simulink model "Quadrotor"  (R2014a)
settings: Solver=ode45  StartTime=0.0  StopTime=10.0  MaxStep=0.1  RelTol=1e-3
InitFcn:
  | parameters;
  | [b, d] = Bemt();
values from neighbouring files (symbols this model uses):
  g = 9.81    [Bemt.m]
  I = diag([0.0086,0.0086,0.0172])    [Bemt.m]
  Iprop = 12*10^-6    (= 1.2e-05)    [Bemt.m]
  Kmot = 1/(1900/60*2*pi)    (= 0.00502594557132)    [Bemt.m]
  L = 0.225    [Bemt.m]
  m = 0.58    [Bemt.m]
  Rmot = 0.128    [Bemt.m]
undefined symbols (not defined in the file or in its folder): attitudeInit, b, d, MotorSpeedInit, omegaInit, posInit, velInit
settings Model: Creator=rudink  LastModifiedBy=daniel
settings DebuggingCC: UnderspecifiedInitializationDetection=Classic  StateNameClashWarn=warning

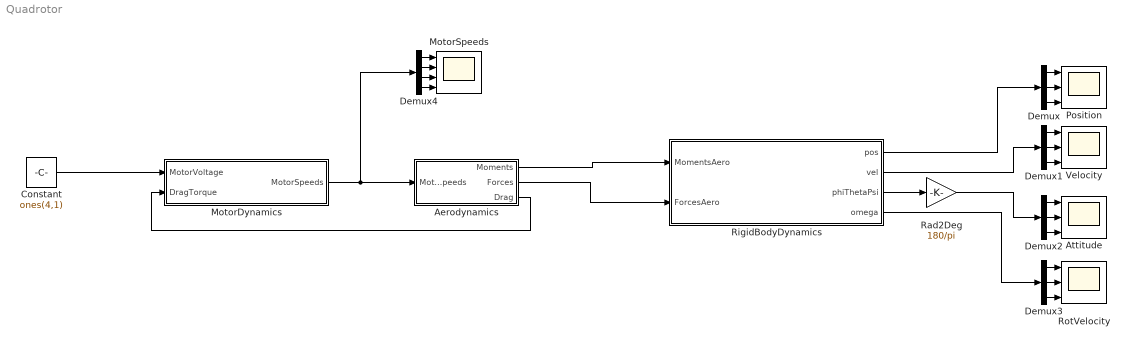
== system Quadrotor ==
  Aerodynamics : Subsystem
  Attitude : Scope  NumInputPorts=3
      settings: YMin=-5~-5~-5  YMax=5~5~5  SaveName=ScopeData2  MaxDataPoints=10000
  Constant : Constant  Value=ones(4,1)
  Demux{,1..3} (4 alike) : Demux  Outputs=3
  Demux4 : Demux
  MotorDynamics : Subsystem
  MotorSpeeds : Scope  NumInputPorts=4
      settings: YMin=-5~-5~-5~-5  YMax=5~5~5~5  SaveName=ScopeData4  MaxDataPoints=10000
  Position : Scope  NumInputPorts=3
      settings: YMin=-5~-5~-5  YMax=5~5~5  MaxDataPoints=10000
  Rad2Deg : Gain  Gain=180/pi
  RigidBodyDynamics : Subsystem
  RotVelocity : Scope  NumInputPorts=3
      settings: YMin=-5~-5~-5  YMax=5~5~5  SaveName=ScopeData3  MaxDataPoints=10000
  Velocity : Scope  NumInputPorts=3
      settings: YMin=-5~-5~-5  YMax=5~5~5  MaxDataPoints=10000
  wires:
  Demux/2 -> Position/2
  Demux/3 -> Position/3
  Demux/1 -> Position/1
  RigidBodyDynamics/1(pos) -> Demux/1
  Demux1/2 -> Velocity/2
  Demux1/3 -> Velocity/3
  Demux1/1 -> Velocity/1
  Demux2/2 -> Attitude/2
  Demux2/3 -> Attitude/3
  Demux2/1 -> Attitude/1
  Demux3/2 -> RotVelocity/2
  Demux3/3 -> RotVelocity/3
  Demux3/1 -> RotVelocity/1
  RigidBodyDynamics/2(vel) -> Demux1/1
  RigidBodyDynamics/3(phiThetaPsi) -> Rad2Deg/1
  RigidBodyDynamics/4(omega) -> Demux3/1
  Aerodynamics/2(Forces) -> RigidBodyDynamics/2(ForcesAero)
  Aerodynamics/1(Moments) -> RigidBodyDynamics/1(MomentsAero)
  Rad2Deg/1 -> Demux2/1
  MotorDynamics/1(MotorSpeeds) -> Demux4/1, Aerodynamics/1(MotorSpeeds)
  Aerodynamics/3(Drag) -> MotorDynamics/2(DragTorque)
  Constant/1 -> MotorDynamics/1(MotorVoltage)
  Demux4/2 -> MotorSpeeds/2
  Demux4/1 -> MotorSpeeds/1
  Demux4/3 -> MotorSpeeds/3
  Demux4/4 -> MotorSpeeds/4

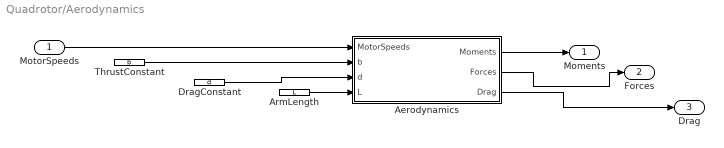
== system Quadrotor/Aerodynamics ==
  MotorSpeeds : Inport
  Aerodynamics : MATLAB Function  TreatAsAtomicUnit=on
  ArmLength : Constant  Value=L
  DragConstant : Constant  Value=d
  ThrustConstant : Constant  Value=b
  Moments : Outport
  Forces : Outport  Port=2
  Drag : Outport  Port=3
  wires:
  Aerodynamics/1(Moments) -> Moments/1
  Aerodynamics/2(Forces) -> Forces/1
  MotorSpeeds/1 -> Aerodynamics/1(MotorSpeeds)
  ThrustConstant/1 -> Aerodynamics/2(b)
  DragConstant/1 -> Aerodynamics/3(d)
  ArmLength/1 -> Aerodynamics/4(L)
  Aerodynamics/3(Drag) -> Drag/1

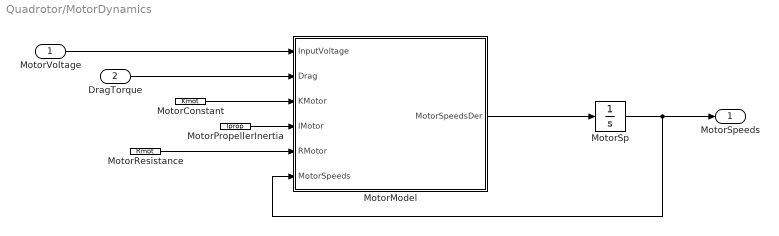
== system Quadrotor/MotorDynamics ==
  MotorVoltage : Inport
  DragTorque : Inport  Port=2
  MotorConstant : Constant  Value=Kmot
  MotorModel : MATLAB Function  TreatAsAtomicUnit=on
  MotorPropellerInertia : Constant  Value=Iprop
  MotorResistance : Constant  Value=Rmot
  MotorSp : Integrator  InitialCondition=MotorSpeedInit
  MotorSpeeds : Outport
  wires:
  MotorVoltage/1 -> MotorModel/1(InputVoltage)
  DragTorque/1 -> MotorModel/2(Drag)
  MotorModel/1(MotorSpeedsDer) -> MotorSp/1
  MotorSp/1 -> MotorModel/6(MotorSpeeds), MotorSpeeds/1
  MotorConstant/1 -> MotorModel/3(KMotor)
  MotorPropellerInertia/1 -> MotorModel/4(IMotor)
  MotorResistance/1 -> MotorModel/5(RMotor)

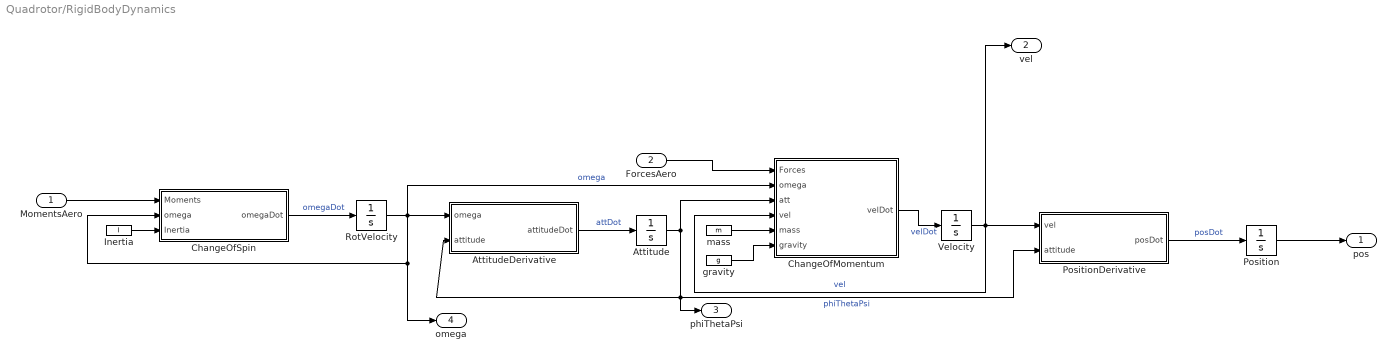
== system Quadrotor/RigidBodyDynamics ==
  MomentsAero : Inport
  ForcesAero : Inport  Port=2
  Attitude : Integrator  InitialCondition=attitudeInit
  AttitudeDerivative : MATLAB Function  TreatAsAtomicUnit=on
  ChangeOfMomentum : MATLAB Function  TreatAsAtomicUnit=on
  ChangeOfSpin : MATLAB Function  TreatAsAtomicUnit=on
  Inertia : Constant  Value=I
  Position : Integrator  InitialCondition=posInit
  PositionDerivative : MATLAB Function  TreatAsAtomicUnit=on
  RotVelocity : Integrator  InitialCondition=omegaInit
  Velocity : Integrator  InitialCondition=velInit
  gravity : Constant  Value=g
  mass : Constant  Value=m
  pos : Outport
  vel : Outport  Port=2
  phiThetaPsi : Outport  Port=3
  omega : Outport  Port=4
  wires:
  MomentsAero/1 -> ChangeOfSpin/1(Moments)
  ChangeOfSpin/1(omegaDot) -> RotVelocity/1  "omegaDot"
  RotVelocity/1 -> ChangeOfMomentum/2(omega), AttitudeDerivative/1(omega), omega/1, ChangeOfSpin/2(omega)  "omega"
  AttitudeDerivative/1(attitudeDot) -> Attitude/1  "attDot"
  Attitude/1 -> ChangeOfMomentum/3(att), phiThetaPsi/1, PositionDerivative/2(attitude), AttitudeDerivative/2(attitude)  "phiThetaPsi"
  ChangeOfMomentum/1(velDot) -> Velocity/1  "velDot"
  Velocity/1 -> vel/1, PositionDerivative/1(vel), ChangeOfMomentum/4(vel)  "vel"
  ForcesAero/1 -> ChangeOfMomentum/1(Forces)
  PositionDerivative/1(posDot) -> Position/1  "posDot"
  Position/1 -> pos/1
  Inertia/1 -> ChangeOfSpin/3(Inertia)
  mass/1 -> ChangeOfMomentum/5(mass)
  gravity/1 -> ChangeOfMomentum/6(gravity)

== matlab function Quadrotor/RigidBodyDynamics/AttitudeDerivative ==
  data: omega input; attitude input; attitudeDot output
function attitudeDot = fcn(omega, attitude)
%Propeller Analysis and Dynamic Modeling I - slide 22
phi = attitude(1);
theta = attitude(2);

Jr = [1, 0        , -sin(theta)        ;
      0, cos(phi) , sin(phi)*cos(theta);
      0, -sin(phi), cos(phi)*cos(theta) ];

attitudeDot = Jr^-1 * omega;

== matlab function Quadrotor/RigidBodyDynamics/ChangeOfSpin ==
  data: Moments input; omegaDot output; omega input; Inertia input
function omegaDot = fcn(Moments, omega, Inertia)
%Propeller Analysis and Dynamic Modeling I - slide 22

omegaDot = Inertia^-1 * (Moments - cross(omega,(Inertia*omega)) );

== matlab function Quadrotor/RigidBodyDynamics/ChangeOfMomentum ==
  data: Forces input; velDot output; omega input; att input; vel input; mass input; gravity input
function velDot = fcn(Forces, omega, att, vel, mass, gravity)
%#codegen
phi = att(1);
theta = att(2);
psi = att(3);

Ceb = [ cos(psi)*cos(theta), cos(psi)*sin(theta)*sin(phi) - sin(psi)*cos(phi), cos(psi)*sin(theta)*cos(phi)+sin(psi)*sin(phi);
        sin(psi)*cos(theta), sin(psi)*sin(theta)*sin(phi) + cos(psi)*cos(phi), sin(psi)*sin(theta)*cos(phi)-cos(psi)*sin(phi);
        -sin(theta),         cos(theta)*sin(phi),                              cos(theta)*cos(phi)                            ];


velDot = ( Forces+Ceb'*[0;0;mass*gravity] - cross(omega,mass*vel) ) / mass;

== matlab function Quadrotor/RigidBodyDynamics/PositionDerivative ==
  data: vel input; attitude input; posDot output
function posDot = fcn(vel, attitude)
%#codegen
phi = attitude(1);
theta = attitude(2);
psi = attitude(3);

Ceb = [ cos(psi)*cos(theta), cos(psi)*sin(theta)*sin(phi) - sin(psi)*cos(phi), cos(psi)*sin(theta)*cos(phi)+sin(psi)*sin(phi);
        sin(psi)*cos(theta), sin(psi)*sin(theta)*sin(phi) + cos(psi)*cos(phi), sin(psi)*sin(theta)*cos(phi)-cos(psi)*sin(phi);
        -sin(theta),         cos(theta)*sin(phi),                              cos(theta)*cos(phi)                            ];

posDot = Ceb*vel;

== matlab function Quadrotor/Aerodynamics/Aerodynamics ==
  data: MotorSpeeds input; Moments output; Forces output; b input; d input; L input; Drag output
function [Moments, Forces, Drag] = fcn(MotorSpeeds,b,d,L)
%#codegen
Drag = d*MotorSpeeds.^2; % Per propeller
Ti = b*MotorSpeeds.^2 ; 
Forces = [0;0;sum( -Ti ) ];
Moments = [0;0;Drag(1)-Drag(2)+Drag(3)-Drag(4)] + ...
   L*[Ti(4)-Ti(2);Ti(1)-Ti(3);0]   ;

== matlab function Quadrotor/MotorDynamics/MotorModel ==
  data: InputVoltage input; Drag input; KMotor input; IMotor input; RMotor input; MotorSpeeds input; MotorSpeedsDer output
function MotorSpeedsDer = fcn(InputVoltage,Drag,KMotor,IMotor,RMotor, MotorSpeeds)
%#codegen
Uind = KMotor * MotorSpeeds;
i = ( InputVoltage - Uind )/RMotor; 
Tm = KMotor*i;


% Calculate the derivative of the motorspeed
MotorSpeedsDer = ( Tm - Drag ) / IMotor ;
